simulink model "MachExtension2Cdtable"  (R2023b)
settings: Solver=VariableStepAuto  StartTime=0.0  StopTime=10.0  RelTol=1e-3
model workspace (MAT data in the model file):
  surfaceBlockParameters1 = Simulink.LookupTable
  surfaceBlockParameters1.Table = Simulink.lookuptable.Table
  surfaceBlockParameters1.Table.Value = [0.717  0.734  0.757  0.783  0.814  0.847  0.883  0.921  0.961  1.003  1.046; 0.465  0.487  0.515  0.548  0.586  0.628  0.672  0.72  0.769  0.821  0.875; 0.4295  0.4534  0.4851  0.5219  0.5637  0.6104  0.6602  0.7128  0.7676  0.8253  0.883; 0.4088  0.4374  0.4738  0.516  0.5652  0.6192  0.6772  0.739  0.803  0.8688  0.9334; 0.3965  0.433  0.484  0.5444  0.6125  0.6869  0.7674  0.8519  0.9401  1.0286  1.1181; 0.4314  0.4746  0.539  0.617  0.667  0.797  0.8976  1.0038  1.1144  1.2244  1.334; 0.5405  0.5835  0.649  0.7275  0.8145  0.91  1.0115  1.119  1.229  1.339  1.449; 0.5088  0.55  0.6132  0.6878  0.7716  0.8624  0.9596  1.0624  1.1668  1.2716  1.3754; 0.4844  0.5234  0.5828  0.6532  0.7319  0.8173  0.9094  1.0058  1.1029  1.2003  1.2974; 0.4628  0.5006  0.5574  0.6244  0.7002  0.7828  0.8706  0.9624  1.055  1.1486  1.2412]
  surfaceBlockParameters1.Table.Dimensions = [10 11]
  surfaceBlockParameters1.Table.DataType = 'auto'
  surfaceBlockParameters1.Table.FieldName = 'Table_zData'
  surfaceBlockParameters1.Breakpoints(1) = Simulink.lookuptable.Breakpoint
  surfaceBlockParameters1.Breakpoints(1).Value = [0.01 0.2 0.39 0.58 0.77 0.96 1.15 1.34 1.53 1.72]
  surfaceBlockParameters1.Breakpoints(1).TunableSizeName = 'N1'
  surfaceBlockParameters1.Breakpoints(1).Dimensions = [1 10]
  surfaceBlockParameters1.Breakpoints(1).DataType = 'auto'
  surfaceBlockParameters1.Breakpoints(1).FieldName = 'BP1_xData'
  surfaceBlockParameters1.Breakpoints(2) = Simulink.lookuptable.Breakpoint
  surfaceBlockParameters1.Breakpoints(2).Value = [0 0.1 0.2 0.3 0.4 0.5 0.6 0.7 0.8 0.9 1]
  surfaceBlockParameters1.Breakpoints(2).TunableSizeName = 'N2'
  surfaceBlockParameters1.Breakpoints(2).Dimensions = [1 11]
  surfaceBlockParameters1.Breakpoints(2).DataType = 'auto'
  surfaceBlockParameters1.Breakpoints(2).FieldName = 'BP2_yData'
  surfaceBlockParameters1.AllowMultipleInstancesOfTypeToHaveDifferentTableBreakpointSizes = 0
  surfaceBlockParameters1.SupportTunableSize = 0
  surfaceBlockParameters1.StructTypeInfo = Simulink.lookuptable.StructTypeInfo
  surfaceBlockParameters1.StructTypeInfo.Name = 'surfaceBlockParameters_type'
  surfaceBlockParameters1.StructTypeInfo.DataScope = 'Auto'
settings Model: Creator=aless  LastModifiedBy=aless

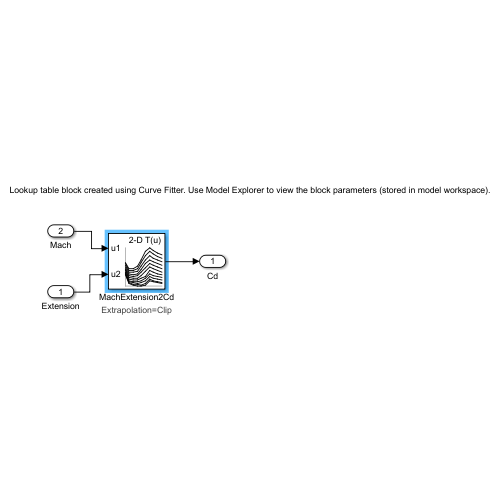
[thumbnail: Simulink's stored preview of the top-level diagram]
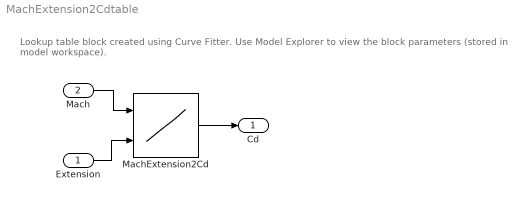
== system MachExtension2Cdtable ==
  note: Lookup table block created using Curve Fitter. Use Model Explorer to view the block parameters (stored in model workspace).
  Extension : Inport
  Mach : Inport  Port=2
  MachExtension2Cd : Lookup_n-D  DataSpecification=Lookup table object  LookupTableObject=surfaceBlockParameters1  BreakpointsForDimension1=[1:3]  BreakpointsForDimension2=[1:3]  ExtrapMethod=Clip  InternalRulePriority=Speed  RndMeth=Simplest
      settings: AttributesFormatString=Extrapolation=%<ExtrapMethod>  InputPortMap=u0,u1
  Cd : Outport
  wires:
  MachExtension2Cd/1 -> Cd/1
  Extension/1 -> MachExtension2Cd/2
  Mach/1 -> MachExtension2Cd/1
